simulink model "EV_0808_mohu"  (R2018a)
settings: Solver=VariableStepAuto  StartTime=0.0  StopTime=1370  RelTol=1e-3
undefined symbols (not defined in the file or in its folder): batt, cyc_spd, cyc_time, DiscIntNeverNeededParam, fr_effi, TIME_STEP, tm, UC, vcu, vehicle
libraries: simulink x9, fuzblock x1
(part 1 of 2)
settings Model: Creator=FlowerCater  LastModifiedBy=FlowerCater
settings SolverCC: ZeroCrossAlgorithm=Adaptive
settings DebuggingCC: MaxConsecutiveZCsMsg=none
settings CodeAppCC: StateflowObjectComments=on

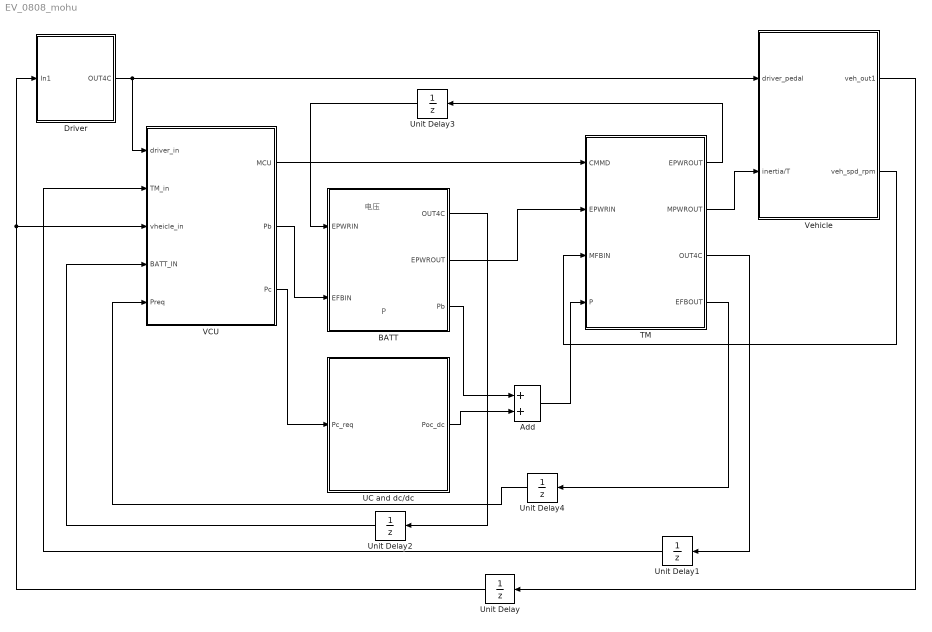
== system EV_0808_mohu ==
  note: 电压
  note: P
  Add : Sum
  BATT : Subsystem
  Driver : Subsystem
  TM : Subsystem
  UC and dc/dc : Subsystem
  Unit Delay : UnitDelay  SampleTime=-1
  Unit Delay1 : UnitDelay  SampleTime=-1
  Unit Delay2 : UnitDelay  SampleTime=-1
  Unit Delay3 : UnitDelay  InitialCondition=590  SampleTime=-1
  Unit Delay4 : UnitDelay  InitialCondition=590  SampleTime=-1
  VCU : Subsystem
  Vehicle : Subsystem
  wires:
  TM/4(EFBOUT) -> Unit Delay4/1
  Unit Delay1/1 -> VCU/2(TM_in)
  Unit Delay2/1 -> VCU/4(BATT_IN)
  TM/2(MPWROUT) -> Vehicle/2(inertia/T)
  TM/1(EPWROUT) -> Unit Delay3/1
  Driver/1(OUT4C) -> VCU/1(driver_in), Vehicle/1(driver_pedal)
  Unit Delay/1 -> Driver/1(In1), VCU/3(vheicle_in)
  Unit Delay3/1 -> BATT/1(EPWRIN)
  BATT/2(EPWROUT) -> TM/2(EPWRIN)
  BATT/1(OUT4C) -> Unit Delay2/1
  VCU/3(Pc) -> UC and dc/dc/1(Pc_req)
  Add/1 -> TM/4(P)
  UC and dc/dc/1(Poc_dc) -> Add/2
  Vehicle/2(veh_spd_rpm) -> TM/3(MFBIN)
  Unit Delay4/1 -> VCU/5(Preq)
  VCU/2(Pb) -> BATT/2(EFBIN)
  VCU/1(MCU) -> TM/1(CMMD)
  BATT/3(Pb) -> Add/1
  TM/3(OUT4C) -> Unit Delay1/1
  Vehicle/1(veh_out1) -> Unit Delay/1

== system EV_0808_mohu/BATT ==
  note: batt_loss_kw
  note: batt_soc
  EPWRIN : Inport
  EFBIN : Inport  Port=2
  Battery degradation : Subsystem
  Bus Creator : BusCreator  Inputs=2
  Bus Creator2 : BusCreator  Inputs=10
  Bus Selector : BusSelector  OutputSignals=V_Volt_v
  Constant2 : Constant  Value=25
  Derice SOC : Subsystem
  Divide1 : Product  Inputs=/*
  Internal Heating : Subsystem
  Product : Product
  Saturation : Saturate  UpperLimit=250  LowerLimit=-200
  batt_curr : Scope
  batt_curra : Scope
  batt_soc : Scope
  batt_v : Scope
  max power limitation : Subsystem
  output voltage : Subsystem
  resistance and voltage : Subsystem
  OUT4C : Outport  InitialOutput=0
  EPWROUT : Outport  Port=2  InitialOutput=0
  Pb : Outport  Port=3
  tag scope: Ub=global
  wires:
  output voltage/2(batt_volt_drop_v) -> Internal Heating/3(lost_volt_v)
  Derice SOC/2(ah_throughout_ahrs) -> resistance and voltage/3(ah_throughout_ahrs), Battery degradation/2(DR), Bus Creator2/9  "batt_throughout_ah"
  output voltage/1(batt_out_volt_v) -> batt_v/1, Bus Creator2/2, [Ub], Bus Creator/1  "V_Volt_v"
  Derice SOC/1(batt_soc) -> Bus Creator2/6, Bus Creator/2, max power limitation/3(batt_soc), Battery degradation/1(SOC), batt_soc/1, resistance and voltage/2(batt_soc)  "batt_soc"
  max power limitation/1(dischar_peak_pwr_kw) -> Bus Creator2/7  "dischar_peak_pwr_kw"
  Bus Creator/1 -> EPWROUT/1
  resistance and voltage/1(batt_oc_volt_v) -> max power limitation/1(batt_volt_oc_v), output voltage/1(battery_oc_volt_v)
  max power limitation/2(char_peak_pwr_kw) -> Bus Creator2/8  "char_peak_pwr_kw"
  Derice SOC/3(batt_curr_amp) -> resistance and voltage/4(current_amp), Bus Creator2/3, Product/2, Saturation/1, Internal Heating/2(Curr_amp), output voltage/2(batt_curr_amp)  "V_Curr_amp"
  Constant2/1 -> Internal Heating/1(amb_temp_degc)
  resistance and voltage/2(batt_res_ohm) -> max power limitation/2(batt_res_ohm), Bus Creator2/5, output voltage/3(battery_res_ohms)  "batt_res_ohm"
  Internal Heating/2(batt_temp_degc) -> resistance and voltage/1(temp_degc), max power limitation/4(batt_temp_degc), Bus Creator2/4  "batt_temp_degc"
  EPWRIN/1 -> Bus Selector/1
  Bus Selector/1 -> Derice SOC/1(EPWRIN), Divide1/1  "<V_Volt_v>"
  Bus Creator2/1 -> OUT4C/1
  Internal Heating/1(batt_pwr_lose_kw) -> Bus Creator2/10
  Saturation/1 -> Product/1, batt_curra/1
  Divide1/1 -> batt_curr/1, Derice SOC/2(EFBIN)
  Product/1 -> Pb/1
  EFBIN/1 -> Divide1/2
  Battery degradation/1(aging) -> Bus Creator2/1

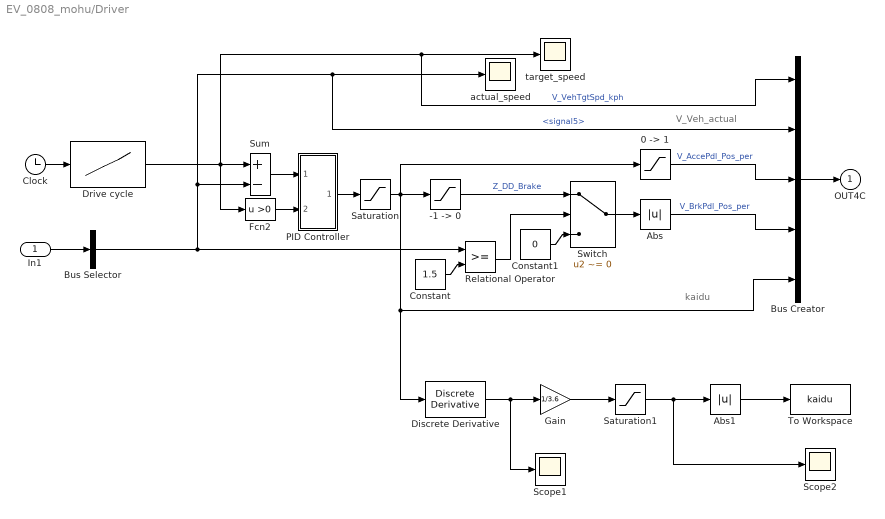
== system EV_0808_mohu/Driver ==
  note: V_Veh_actual
  note: kaidu
  In1 : Inport
  "-1 -> 0" : Saturate  UpperLimit=0  LowerLimit=-1
  "0 -> 1 " : Saturate  UpperLimit=1  LowerLimit=0
  Abs : Abs  SaturateOnIntegerOverflow=on
  Abs1 : Abs
  Bus Creator : BusCreator  Inputs=5
  Bus Selector : BusSelector  OutputSignals=signal5
  Clock : Clock
  Constant : Constant  Value=1.5
  Constant1 : Constant  Value=0
  Discrete Derivative : simulink/Discrete/Discrete Derivative  gainval=1.0  ICPrevScaledInput=0.0  OutMin=[]  OutMax=[]  OutDataType=fixdt(1, 16)  OutScaling=2^-10  DoSatur=off
  "Drive cycle " : Lookup  InputValues=cyc_time  Table=cyc_spd  SaturateOnIntegerOverflow=on
  Fcn2 : Fcn  Expr=u >0
  Gain : Gain  Gain=1/3.6
  PID Controller : Subsystem  mask(PID Controller){P=1, I=0.001, D=0, initial=0, max=1, min=-1}
      mask prompts: P "Proportional:"; I "Integral:"; D "Derivative:"; initial "Initial value"; max "Range max value"; min "Range min value"
      mask help:
      | Enter expressions for proportional, integral, and derivative terms.
      | P+I/s+Ds
      mask Help: This block implements a PID controller where parameters are entered for the Proportional, Integral and Derivative terms. Unmask this block to see how it works. The derivative term is implemented using a true derivative block.
      mask Display: disp('PID')
  Relational Operator : RelationalOperator  OutDataTypeStr=boolean  RndMeth=Nearest
  Saturation : Saturate  UpperLimit=1  LowerLimit=-1
  Saturation1 : Saturate  UpperLimit=1  LowerLimit=-1
  Scope1 : Scope
  Scope2 : Scope
  Sum : Sum  Inputs=+-  SaturateOnIntegerOverflow=on
  Switch : Switch  Criteria=u2 ~= 0
  To Workspace : ToWorkspace  VariableName=kaidu  SaveFormat=Timeseries  SampleTime=-1
  actual_speed : Scope
  target_speed : Scope
  OUT4C : Outport  InitialOutput=0
  wires:
  Bus Creator/1 -> OUT4C/1
  Fcn2/1 -> PID Controller/2(reset)
  Bus Selector/1 -> Bus Creator/2, actual_speed/1, Sum/2, Relational Operator/1  "<signal5>"
  Sum/1 -> PID Controller/1(In_1)
  Constant/1 -> Relational Operator/2
  Relational Operator/1 -> Switch/2
  Constant1/1 -> Switch/3
  PID Controller/1(Out_1) -> Saturation/1
  Switch/1 -> Abs/1
  "-1 -> 0"/1 -> Switch/1  "Z_DD_Brake"
  Clock/1 -> "Drive cycle "/1
  "Drive cycle "/1 -> Fcn2/1, Bus Creator/1, target_speed/1, Sum/1  "V_VehTgtSpd_kph"
  Saturation/1 -> "-1 -> 0"/1, "0 -> 1 "/1, Bus Creator/5, Discrete Derivative/1
  Abs/1 -> Bus Creator/4  "V_BrkPdl_Pos_per"
  "0 -> 1 "/1 -> Bus Creator/3  "V_AccePdl_Pos_per"
  In1/1 -> Bus Selector/1
  Discrete Derivative/1 -> Scope1/1, Gain/1
  Abs1/1 -> To Workspace/1
  Saturation1/1 -> Scope2/1, Abs1/1
  Gain/1 -> Saturation1/1

== system EV_0808_mohu/TM ==
  note: 电池动力输入
  note: 电机转动惯量
  CMMD : Inport
  EPWRIN : Inport  Port=2
  MFBIN : Inport  Port=3
  P : Inport  Port=4
  Bus Creator : BusCreator  Inputs=5
  Bus Creator1 : BusCreator  Inputs=1
  Bus Creator2 : BusCreator  Inputs=2
  Bus Selector : BusSelector  OutputSignals=V_BrkTq_Req_nm
  Bus Selector1 : BusSelector  OutputSignals=signal1
  Bus Selector2 : BusSelector  OutputSignals=V_Volt_v,batt_soc
  Constant : Constant  Value=tm.inertia
  Current Generation : Subsystem
  Intenal Heating : Subsystem
  Terminator : Terminator
  Terminator1 : Terminator
  Torque management : Subsystem
  Unit Delay1 : UnitDelay  SampleTime=-1
  EPWROUT : Outport
  MPWROUT : Outport  Port=2
  OUT4C : Outport  Port=3
  EFBOUT : Outport  Port=4
  wires:
  Constant/1 -> Bus Creator2/2  "tm.inertia"
  Current Generation/2(motor_eff_per) -> Terminator/1
  Torque management/1(" torque_req_nm") -> Bus Creator/4, Bus Creator2/1, Current Generation/1(torque_req_nm)  "V_Actual_BrkTq_nm"
  Current Generation/3(pwr_loss_w) -> Bus Creator/5, Intenal Heating/1(pwr_loss_w)  "TM_loss_W"
  EPWRIN/1 -> Bus Selector2/1
  CMMD/1 -> Bus Selector/1
  Bus Selector/1 -> Torque management/1(tq_req_nm)  "<V_BrkTq_Req_nm>"
  Bus Creator2/1 -> MPWROUT/1
  MFBIN/1 -> Unit Delay1/1
  Current Generation/1(motor_curr_amp) -> Bus Creator/3  "V_CurrDCamp"
  Intenal Heating/1(cool_temp_degc) -> Bus Creator/1, Torque management/3(cool_temp_degc)  "V_Cool_Temp_degc"
  Bus Creator/1 -> OUT4C/1
  Unit Delay1/1 -> Bus Selector1/1
  Bus Selector1/1 -> Current Generation/2(motor_spd_rpm), Torque management/4(motor_spd_rpm), Bus Creator/2  "<signal1>"
  Bus Selector2/1 -> Current Generation/3(volt_v), Bus Creator1/1  "<V_Volt_v>"
  Bus Creator1/1 -> EPWROUT/1
  Bus Selector2/2 -> Torque management/2(soc)  "<batt_soc>"
  Current Generation/4(P) -> EFBOUT/1  "p"
  P/1 -> Terminator1/1

== system EV_0808_mohu/UC and dc//dc ==
  Pc_req : Inport
  Gain : Gain  Gain=-1
  Memory : Memory
  Pcdc : Scope
  Product1 : Product
  Switch : Switch  Criteria=u2 > Threshold
  UC : Subsystem
  charge : Lookup_n-D  BreakpointsForDimension1=[0:2000:8000]  BreakpointsForDimension2=[0.2:0.2:1]  Table=[0.8 0.8 0.8 0.8 0.8;0.945 0.952 0.965 0.972 0.977;0.94 0.95 0.957 0.965 0.97;0.938 0.946 0.952 0.962 0.964;0.934 0.944 0.95 0.96 0.962]  InternalRulePriority=Speed  RndMeth=Simplest  InputSameDT=on
  discharge : Lookup_n-D  BreakpointsForDimension1=[0:2000:8000]  BreakpointsForDimension2=[0.2:0.2:1]  Table=[0.8 0.8 0.8 0.8 0.8;0.945 0.952 0.965 0.972 0.977;0.94 0.95 0.957 0.965 0.97;0.938 0.946 0.952 0.962 0.964;0.934 0.944 0.95 0.96 0.962]  InternalRulePriority=Speed  RndMeth=Simplest  InputSameDT=on
  电压比 : Product  Inputs=/*
  电压比1 : Product  Inputs=*/
  Poc_dc : Outport
  wires:
  电压比1/1 -> Switch/1
  电压比/1 -> Memory/1
  UC/1(Pc) -> 电压比1/1, Product1/1, Switch/2, discharge/1, Gain/1
  charge/1 -> Product1/2
  discharge/1 -> 电压比1/2
  Gain/1 -> charge/1
  [Uc] -> 电压比/1
  Product1/1 -> Switch/3
  Memory/1 -> discharge/2, charge/2
  [Ub] -> 电压比/2
  Switch/1 -> Pcdc/1, Poc_dc/1
  Pc_req/1 -> UC/1(Pc-req (W))

== system EV_0808_mohu/VCU ==
  driver_in : Inport
  TM_in : Inport  Port=2
  vheicle_in : Inport  Port=3
  BATT_IN : Inport  Port=4
  Preq : Inport  Port=5
  Bus Creator2 : BusCreator  Inputs=5
  Display : Display
  Gain : Gain
  Gain1 : Gain
  Gain2 : Gain
  Subsystem1 : Subsystem
  Subsystem3 : Subsystem
  To Workspace : ToWorkspace  VariableName=tm_act_tq11  SampleTime=-1
      settings: MaxDataPoints=Inf
  To Workspace1 : ToWorkspace  VariableName=tm_act_spd  SampleTime=-1
      settings: MaxDataPoints=Inf
  controller : Subsystem
  max generation  torque : Lookup  InputValues=tm.max_gen_tq_x_rpm  Table=tm.max_gen_tq_y_nm  LookUpMeth=Interpolation-Use End Values
  max motoring torque : Lookup  InputValues=tm.max_mot_tq_x_rpm  Table=tm.max_mot_tq_y_nm  LookUpMeth=Interpolation-Use End Values
  续驶里程估计 : Subsystem
  能耗计算 : Subsystem
  MCU : Outport
  Pb : Outport  Port=2
  Pc : Outport  Port=3
  wires:
  Gain/1 -> Bus Creator2/1  "V_BrkTq_Req_nm"
  max motoring torque/1 -> Bus Creator2/2  "V_MaxMotTq_nm"
  max generation  torque/1 -> Bus Creator2/3  "V_MaxGenTq_nm"
  Gain1/1 -> Bus Creator2/4, To Workspace1/1  "V_Spd_rpm"
  Gain2/1 -> Bus Creator2/5, To Workspace/1  "V_ActBrkTq_nm"
  Bus Creator2/1 -> MCU/1
  Subsystem1/1(V_Spd_rmp) -> Subsystem3/1(V_Spd_rpm), max motoring torque/1, Gain1/1, max generation  torque/1
  TM_in/1 -> 能耗计算/2(In3), Subsystem1/1(TM_in)
  driver_in/1 -> 能耗计算/1(In1), Subsystem1/2(Dri_in)
  vheicle_in/1 -> 续驶里程估计/2(veh_in), Subsystem1/3(vheicle_in), 能耗计算/3(In2)
  BATT_IN/1 -> 续驶里程估计/1(batt_in), 能耗计算/4(In4)
  Subsystem1/2(rotor drive torque available nm) -> Gain2/1
  Subsystem3/1(TM_TqReq_nm) -> Gain/1
  Subsystem1/3(Tq_Req_nm) -> Subsystem3/2(dri_TqReq_nm)
  能耗计算/1(E_FS) -> Display/1
  Preq/1 -> controller/1(Preq (W))
  controller/1(Pb (W)) -> Pb/1
  controller/2(Pc (W)) -> Pc/1

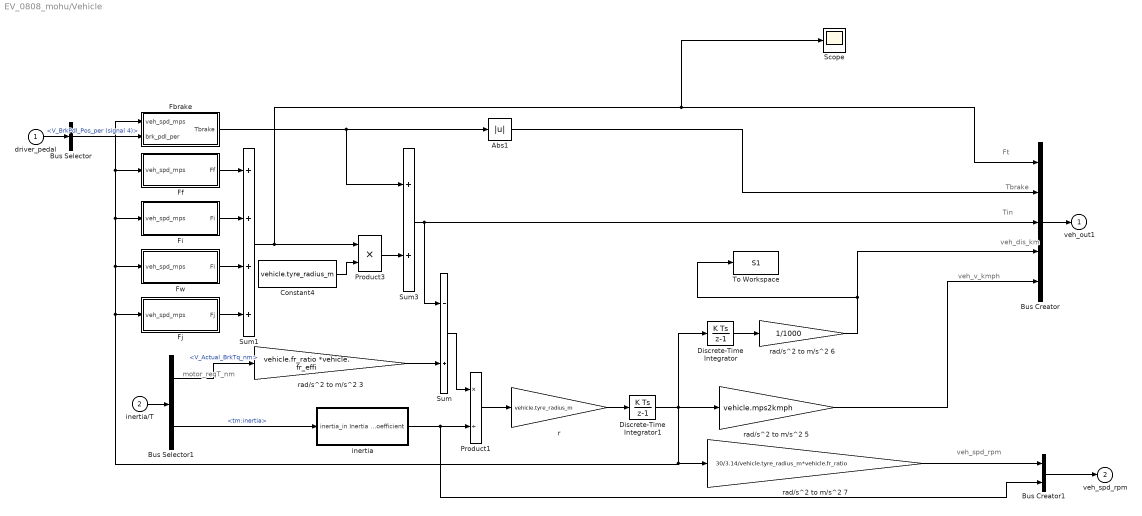
== system EV_0808_mohu/Vehicle ==
  note: veh_spd_rpm
  note: veh_v_kmph
  note: veh_dis_km
  note: Tin
  note: Tbrake
  note: Ft
  note: motor_reqT_nm
  driver_pedal : Inport
  inertia/T : Inport  Port=2
  Abs1 : Abs
  Bus Creator : BusCreator  Inputs=5
  Bus Creator1 : BusCreator  Inputs=2
  Bus Selector : BusSelector  OutputSignals=V_BrkPdl_Pos_per (signal 4)
  Bus Selector1 : BusSelector  OutputSignals=V_Actual_BrkTq_nm,tm:inertia
  Constant4 : Constant  Value=vehicle.tyre_radius_m
  Discrete-Time Integrator : DiscreteIntegrator  SampleTime=0.01  ICPrevOutput=DiscIntNeverNeededParam  ICPrevScaledInput=DiscIntNeverNeededParam
  Discrete-Time Integrator1 : DiscreteIntegrator  SampleTime=0.01  LimitOutput=on  LowerSaturationLimit=0  ICPrevOutput=DiscIntNeverNeededParam  ICPrevScaledInput=DiscIntNeverNeededParam
  Fbrake : Subsystem
  Ff : Subsystem
  Fi : Subsystem
  Fj : Subsystem
  Fw : Subsystem
  Product1 : Product  Inputs=*/  SaturateOnIntegerOverflow=on  OutDataTypeStr=Inherit: Same as first input
  Product3 : Product  SaturateOnIntegerOverflow=on  InputSameDT=on  OutDataTypeStr=Inherit: Same as first input
  Scope : Scope
  Sum : Sum  Inputs=-+  SaturateOnIntegerOverflow=on
  Sum1 : Sum  Inputs=++++  SaturateOnIntegerOverflow=on  InputSameDT=on  OutDataTypeStr=Inherit: Same as first input
  Sum3 : Sum  SaturateOnIntegerOverflow=on  InputSameDT=on  OutDataTypeStr=Inherit: Same as first input
  To Workspace : ToWorkspace  VariableName=S1  SampleTime=-1
  inertia : Subsystem
  r : Gain  Gain=vehicle.tyre_radius_m  SaturateOnIntegerOverflow=on  OutDataTypeStr=Inherit: Same as input  ParamDataTypeStr=Inherit: Same as input
  rad/s^2 to m/s^2 3 : Gain  Gain=vehicle.fr_ratio *vehicle. fr_effi  SaturateOnIntegerOverflow=on  OutDataTypeStr=Inherit: Same as input  ParamDataTypeStr=Inherit: Same as input
  rad/s^2 to m/s^2 5 : Gain  Gain=vehicle.mps2kmph  SaturateOnIntegerOverflow=on  OutDataTypeStr=Inherit: Same as input  ParamDataTypeStr=Inherit: Same as input
  rad/s^2 to m/s^2 6 : Gain  Gain=1/1000  SaturateOnIntegerOverflow=on  OutDataTypeStr=Inherit: Same as input  ParamDataTypeStr=Inherit: Same as input
  rad/s^2 to m/s^2 7 : Gain  Gain=30/3.14/vehicle.tyre_radius_m*vehicle.fr_ratio  SaturateOnIntegerOverflow=on  OutDataTypeStr=Inherit: Same as input  ParamDataTypeStr=Inherit: Same as input
  veh_out1 : Outport  InitialOutput=0
  veh_spd_rpm : Outport  Port=2  InitialOutput=0
  wires:
  driver_pedal/1 -> Bus Selector/1
  Ff/1(Ff) -> Sum1/1
  Fi/1(Fi) -> Sum1/2
  Fw/1(Fi) -> Sum1/3
  Fj/1(Fj) -> Sum1/4
  Sum1/1 -> Scope/1, Bus Creator/1, Product3/1
  Constant4/1 -> Product3/2
  Product3/1 -> Sum3/2
  Fbrake/1(Tbrake) -> Abs1/1, Sum3/1
  Abs1/1 -> Bus Creator/2
  rad/s^2 to m/s^2 3/1 -> Sum/2
  Sum3/1 -> Bus Creator/3, Sum/1
  Bus Selector/1 -> Fbrake/2(brk_pdl_per)  "<V_BrkPdl_Pos_per (signal 4)>"
  inertia/1(Inertia coefficient) -> Bus Creator1/2, Product1/2
  Sum/1 -> Product1/1
  Product1/1 -> r/1
  r/1 -> Discrete-Time Integrator1/1
  Bus Selector1/2 -> inertia/1(inertia_in)  "<tm:inertia>"
  Discrete-Time Integrator1/1 -> Fbrake/1(veh_spd_mps), Ff/1(veh_spd_mps), Fi/1(veh_spd_mps), Fw/1(veh_spd_mps), Fj/1(veh_spd_mps), rad/s^2 to m/s^2 7/1, Discrete-Time Integrator/1, rad/s^2 to m/s^2 5/1
  rad/s^2 to m/s^2 5/1 -> Bus Creator/5
  rad/s^2 to m/s^2 7/1 -> Bus Creator1/1
  rad/s^2 to m/s^2 6/1 -> Bus Creator/4, To Workspace/1
  Discrete-Time Integrator/1 -> rad/s^2 to m/s^2 6/1
  inertia/T/1 -> Bus Selector1/1
  Bus Creator/1 -> veh_out1/1
  Bus Creator1/1 -> veh_spd_rpm/1
  Bus Selector1/1 -> rad/s^2 to m/s^2 3/1  "<V_Actual_BrkTq_nm>"

== system EV_0808_mohu/BATT/Battery degradation ==
  note: 额定容量
  SOC : Inport
  DR : Inport  Port=2
  Add3 : Sum  Inputs=++++
  Constant1 : Constant  Value=120
  Constant3 : Constant  Value=0.069
  Constant4 : Constant  Value=21.714
  Divide : Product  Inputs=*/
  Fcn : Fcn  Expr=-0.573*u+0.004*(u^2)
  Fcn1 : Fcn  Expr=3.13*u-2.34*(u^2)
  Product1 : Product  Inputs=3
  aging : Outport
  wires:
  SOC/1 -> Product1/1, Fcn/1
  Divide/1 -> Product1/3, Fcn1/1
  Constant4/1 -> Add3/4
  Fcn1/1 -> Add3/3
  Fcn/1 -> Add3/1
  Product1/1 -> Add3/2
  Constant3/1 -> Product1/2
  Add3/1 -> aging/1
  Constant1/1 -> Divide/2
  DR/1 -> Divide/1

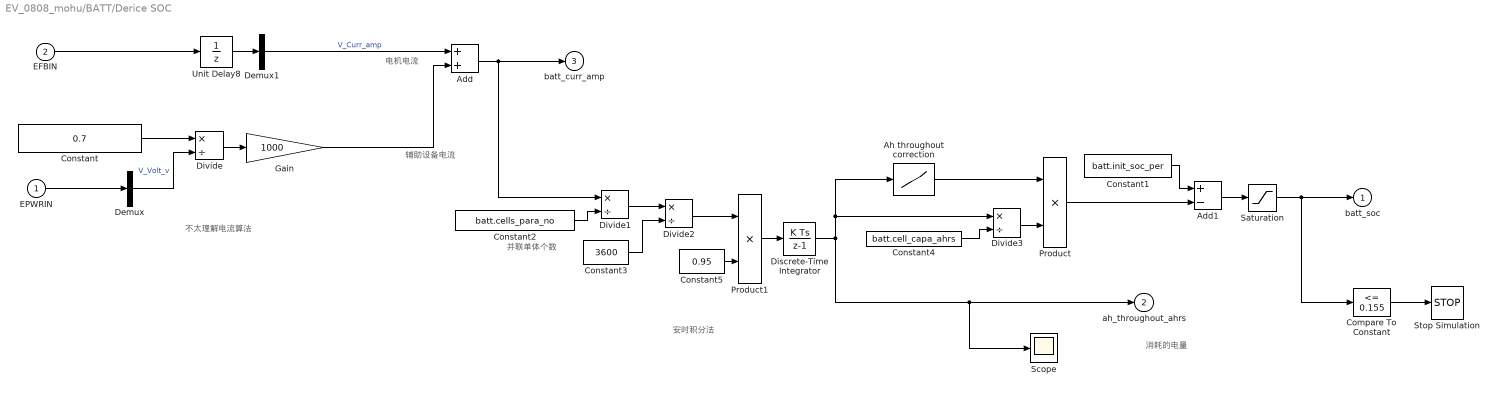
== system EV_0808_mohu/BATT/Derice SOC ==
  note: 安时积分法
  note: 消耗的电量
  note: 并联单体个数
  note: 不太理解电流算法
  note: 辅助设备电流
  note: 电机电流
  EPWRIN : Inport
  EFBIN : Inport  Port=2
  Add : Sum
  Add1 : Sum  Inputs=+-
  Ah throughout correction : Lookup  InputValues=batt.energy_deter_x_brkthrough_ahrs  Table=batt.energy_deter_y  LookUpMeth=Interpolation-Use End Values
  Compare To Constant : simulink/Logic and Bit Operations/Compare To Constant  relop=<=  const=0.155  OutDataTypeStr=boolean
  Constant : Constant  Value=0.7
  Constant1 : Constant  Value=batt.init_soc_per
  Constant2 : Constant  Value=batt.cells_para_no
  Constant3 : Constant  Value=3600
  Constant4 : Constant  Value=batt.cell_capa_ahrs
  Constant5 : Constant  Value=0.95
  Demux : Demux  Outputs=1
  Demux1 : Demux  Outputs=1
  Discrete-Time Integrator : DiscreteIntegrator  SampleTime=0.01  ICPrevOutput=DiscIntNeverNeededParam  ICPrevScaledInput=DiscIntNeverNeededParam
  Divide{,1..3} (4 alike) : Product  Inputs=*/
  Gain : Gain  Gain=1000
  Product : Product
  Product1 : Product
  Saturation : Saturate  UpperLimit=1  LowerLimit=0
  Scope : Scope
  Stop Simulation : Stop
  Unit Delay8 : UnitDelay  SampleTime=-1
  batt_soc : Outport  InitialOutput=0
  ah_throughout_ahrs : Outport  Port=2  InitialOutput=0
  batt_curr_amp : Outport  Port=3  InitialOutput=0
  wires:
  Product/1 -> Add1/2
  Constant1/1 -> Add1/1
  Divide3/1 -> Product/2
  Ah throughout correction/1 -> Product/1
  Add1/1 -> Saturation/1
  EFBIN/1 -> Unit Delay8/1
  Unit Delay8/1 -> Demux1/1
  Constant/1 -> Divide/1
  Demux/1 -> Divide/2  "V_Volt_v"
  EPWRIN/1 -> Demux/1
  Demux1/1 -> Add/1  "V_Curr_amp"
  Gain/1 -> Add/2
  Divide/1 -> Gain/1
  Constant2/1 -> Divide1/2
  Constant3/1 -> Divide2/2
  Constant4/1 -> Divide3/2
  Divide1/1 -> Divide2/1
  Discrete-Time Integrator/1 -> Ah throughout correction/1, Divide3/1, Scope/1, ah_throughout_ahrs/1
  Divide2/1 -> Product1/1
  Constant5/1 -> Product1/2
  Add/1 -> Divide1/1, batt_curr_amp/1
  Product1/1 -> Discrete-Time Integrator/1
  Saturation/1 -> Compare To Constant/1, batt_soc/1
  Compare To Constant/1 -> Stop Simulation/1

== system EV_0808_mohu/BATT/Internal Heating ==
  note: 电池损失功率
  amb_temp_degc : Inport
  Curr_amp : Inport  Port=2
  lost_volt_v : Inport  Port=3
  1/thermal capacity : Gain  Gain=1/(batt.thermal_capa_jpk*batt.cells_para_no*batt.cells_series_no)  SaturateOnIntegerOverflow=on  OutDataTypeStr=Inherit: Same as input  ParamDataTypeStr=Inherit: Same as input
  1/thermal resistance : Gain  Gain=batt.thermal_disp_wpk  SaturateOnIntegerOverflow=on  OutDataTypeStr=Inherit: Same as input  ParamDataTypeStr=Inherit: Same as input
  Abs : Abs  SaturateOnIntegerOverflow=on
  Discrete-Time Integrator1 : DiscreteIntegrator  SampleTime=0.01  LimitOutput=on  LowerSaturationLimit=0  ICPrevOutput=DiscIntNeverNeededParam  ICPrevScaledInput=DiscIntNeverNeededParam
  Gain1 : Gain  Gain=1/1000
  Product1 : Product  SaturateOnIntegerOverflow=on  InputSameDT=on  OutDataTypeStr=Inherit: Same as first input
  Sum1 : Sum  Inputs=+-  SaturateOnIntegerOverflow=on  InputSameDT=on  OutDataTypeStr=Inherit: Same as first input
  Sum2 : Sum  Inputs=+-  SaturateOnIntegerOverflow=on  InputSameDT=on  OutDataTypeStr=Inherit: Same as first input
  To Workspace : ToWorkspace  VariableName=batt_temp_degc  SaveFormat=Timeseries  SampleTime=-1
  batt_pwr_lose_kw : Outport  InitialOutput=0
  batt_temp_degc : Outport  Port=2  InitialOutput=0
  wires:
  Gain1/1 -> batt_pwr_lose_kw/1
  Sum2/1 -> 1/thermal resistance/1
  amb_temp_degc/1 -> Sum2/2
  Product1/1 -> Abs/1
  Abs/1 -> Gain1/1, Sum1/1
  Sum1/1 -> 1/thermal capacity/1
  1/thermal resistance/1 -> Sum1/2
  Curr_amp/1 -> Product1/1
  lost_volt_v/1 -> Product1/2
  1/thermal capacity/1 -> Discrete-Time Integrator1/1
  Discrete-Time Integrator1/1 -> To Workspace/1, batt_temp_degc/1, Sum2/1

== system EV_0808_mohu/BATT/max power limitation ==
  note: 负值取小
  note: 正值取大
  note: 实际充电峰值功率
  note: 实际放电峰值功率
  note: 充电峰值功率
  note: 放电峰值功率
  batt_volt_oc_v : Inport
  batt_res_ohm : Inport  Port=2
  batt_soc : Inport  Port=3
  batt_temp_degc : Inport  Port=4
  MinMax1 : MinMax  Inputs=2  SaturateOnIntegerOverflow=on  InputSameDT=on
  MinMax2 : MinMax  Function=max  Inputs=2  SaturateOnIntegerOverflow=on  InputSameDT=on
  Pack Peak Discharging Power : Lookup2D  RowIndex=batt.max_discharge_pwr_x_soc_per  ColumnIndex=batt.max_discharge_pwr_y_temp_degc  Table=batt.max_discharge_pwr_z_kw  LookUpMeth=Interpolation-Use End Values  SaturateOnIntegerOverflow=on  InputSameDT=on
  Pack peak charging power : Lookup2D  RowIndex=batt.max_charge_pwr_x_soc_per  ColumnIndex=batt.max_charge_pwr_y_temp_degc  Table=batt.max_charge_pwr_z_kw  LookUpMeth=Interpolation-Use End Values  SaturateOnIntegerOverflow=on  InputSameDT=on
  peak chrg power : Subsystem
  peak dischrg power : Subsystem
  dischar_peak_pwr_kw : Outport
  char_peak_pwr_kw : Outport  Port=2
  wires:
  peak chrg power/1(chrg_peak_pwr_kw) -> MinMax2/2
  batt_res_ohm/1 -> peak chrg power/1(batt_res_ohms), peak dischrg power/1(batt_res_ohms)
  MinMax2/1 -> char_peak_pwr_kw/1
  MinMax1/1 -> dischar_peak_pwr_kw/1
  Pack Peak Discharging Power/1 -> MinMax1/1
  Pack peak charging power/1 -> MinMax2/1  "Charge acceptance (<0)"
  peak dischrg power/1(dischrg_peak_pwr_kw) -> MinMax1/2
  batt_volt_oc_v/1 -> peak chrg power/2(batt_oc_volt_v), peak dischrg power/2(batt_oc_volt_v)
  batt_soc/1 -> Pack Peak Discharging Power/1, Pack peak charging power/1
  batt_temp_degc/1 -> Pack Peak Discharging Power/2, Pack peak charging power/2

== system EV_0808_mohu/BATT/output voltage ==
  note: 损失电压
  note: 输出端电压
  battery_oc_volt_v : Inport
  batt_curr_amp : Inport  Port=2
  battery_res_ohms : Inport  Port=3
  Add : Sum  Inputs=+-
  Product : Product
  batt_out_volt_v : Outport  InitialOutput=0
  batt_volt_drop_v : Outport  Port=2  InitialOutput=0
  wires:
  batt_curr_amp/1 -> Product/2
  Product/1 -> batt_volt_drop_v/1, Add/2
  battery_oc_volt_v/1 -> Add/1
  battery_res_ohms/1 -> Product/1
  Add/1 -> batt_out_volt_v/1

== system EV_0808_mohu/BATT/resistance and voltage ==
  note: 根据电量消耗对内阻的修正
  note: 欧姆内阻
  note: 放电电流为正
  note: 电池开路电压
  temp_degc : Inport
  batt_soc : Inport  Port=2
  ah_throughout_ahrs : Inport  Port=3
  current_amp : Inport  Port=4
  Add : Sum
  Constant : Constant  Value=1.0
  Constant1 : Constant  Value=0
  N_series : Gain  Gain=batt.cells_series_no  SaturateOnIntegerOverflow=on  OutDataTypeStr=Inherit: Same as input  ParamDataTypeStr=Inherit: Same as input
  N_series/ N_parallel : Gain  Gain=batt.cells_series_no/batt.cells_para_no  SaturateOnIntegerOverflow=on  OutDataTypeStr=Inherit: Same as input  ParamDataTypeStr=Inherit: Same as input
  Open Circuit Voltage : Lookup2D  RowIndex=batt.cell_open_volt_x_soc_per  ColumnIndex=batt.cell_open_volt_y_degc  Table=batt.cell_open_volt_z_v  LookUpMeth=Interpolation-Use End Values  SaturateOnIntegerOverflow=on  InputSameDT=on
  Product : Product  SaturateOnIntegerOverflow=on  InputSameDT=on  OutDataTypeStr=Inherit: Same as first input
  Product1 : Product
  Relational Operator : RelationalOperator  OutDataTypeStr=boolean  RndMeth=Nearest
  Switch : Switch  Criteria=u2 ~= 0
  To Workspace : ToWorkspace  VariableName=Pd1  SampleTime=-1
  ah throughout correction : Lookup  InputValues=batt.resis_deter_x_brkthrough_ahrs  Table=batt.resis_deter_y  LookUpMeth=Interpolation-Use End Values
  charge resistance table : Lookup2D  RowIndex=batt.resis_chrg_x_soc_per  ColumnIndex=batt.resis_chrg_y_temp_degc  Table=batt.resis_chrg_z_ohm  LookUpMeth=Interpolation-Use End Values  SaturateOnIntegerOverflow=on  InputSameDT=on
  discharge resistance table : Lookup2D  RowIndex=batt.resis_dischrg_x_soc_per  ColumnIndex=batt.resis_dischrg_y_temp_degc  Table=batt.resis_dischrg_z_ohm  LookUpMeth=Interpolation-Use End Values  SaturateOnIntegerOverflow=on  InputSameDT=on
  batt_oc_volt_v : Outport  InitialOutput=0
  batt_res_ohm : Outport  Port=2  InitialOutput=0
  wires:
  Add/1 -> Product/2
  Constant/1 -> Add/2
  ah throughout correction/1 -> Add/1
  ah_throughout_ahrs/1 -> ah throughout correction/1
  Product/1 -> batt_res_ohm/1
  N_series/ N_parallel/1 -> Product/1
  discharge resistance table/1 -> Switch/1
  N_series/1 -> Product1/1, batt_oc_volt_v/1
  Open Circuit Voltage/1 -> N_series/1
  batt_soc/1 -> Open Circuit Voltage/1, discharge resistance table/1, charge resistance table/1
  temp_degc/1 -> Open Circuit Voltage/2, discharge resistance table/2, charge resistance table/2
  current_amp/1 -> Product1/2, Relational Operator/1
  Constant1/1 -> Relational Operator/2
  Relational Operator/1 -> Switch/2
  charge resistance table/1 -> Switch/3
  Switch/1 -> N_series/ N_parallel/1
  Product1/1 -> To Workspace/1

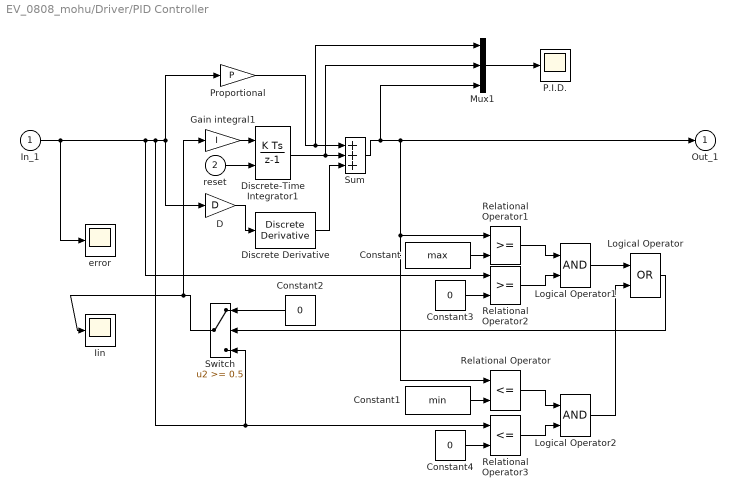
== system EV_0808_mohu/Driver/PID Controller ==
  In_1 : Inport
  reset : Inport  Port=2
  Constant : Constant  Value=max
  Constant1 : Constant  Value=min
  Constant2 : Constant  Value=0
  Constant3 : Constant  Value=0
  Constant4 : Constant  Value=0
  D : Gain  Gain=D  SaturateOnIntegerOverflow=on  OutDataTypeStr=Inherit: Same as input  ParamDataTypeStr=Inherit: Same as input
  Discrete Derivative : simulink/Discrete/Discrete Derivative  gainval=1.0  ICPrevScaledInput=0.0  InputProcessing=Inherited  OutMin=[]  OutMax=[]  OutDataType=fixdt(1, 16)  OutScaling=2^-10  DoSatur=off
  Discrete-Time Integrator1 : DiscreteIntegrator  InitialConditionSource=external  SampleTime=0.01  LimitOutput=on  LowerSaturationLimit=0  ICPrevOutput=DiscIntNeverNeededParam  ICPrevScaledInput=DiscIntNeverNeededParam
  Gain integral1 : Gain  Gain=I  SaturateOnIntegerOverflow=on  OutDataTypeStr=Inherit: Same as input  ParamDataTypeStr=Inherit: Same as input
  Iin : Scope
  Logical Operator : Logic  Operator=OR
  Logical Operator1 : Logic
  Logical Operator2 : Logic
  Mux1 : Mux  Inputs=3
  P.I.D. : Scope
  Proportional : Gain  Gain=P  SaturateOnIntegerOverflow=on  OutDataTypeStr=Inherit: Same as input  ParamDataTypeStr=Inherit: Same as input
  Relational Operator : RelationalOperator  Operator=<=  RndMeth=Nearest  InputSameDT=on
  Relational Operator1 : RelationalOperator  RndMeth=Nearest  InputSameDT=on
  Relational Operator2 : RelationalOperator  RndMeth=Nearest  InputSameDT=on
  Relational Operator3 : RelationalOperator  Operator=<=  RndMeth=Nearest  InputSameDT=on
  Sum : Sum  Inputs=+++  SaturateOnIntegerOverflow=on  InputSameDT=on  OutDataTypeStr=Inherit: Same as first input
  Switch : Switch  Threshold=0.5  SaturateOnIntegerOverflow=on  InputSameDT=on
  error : Scope
  Out_1 : Outport  InitialOutput=0
  wires:
  Logical Operator1/1 -> Logical Operator/1
  Logical Operator2/1 -> Logical Operator/2
  Relational Operator3/1 -> Logical Operator2/2
  Constant4/1 -> Relational Operator3/2
  Relational Operator/1 -> Logical Operator2/1
  Relational Operator2/1 -> Logical Operator1/2
  Constant3/1 -> Relational Operator2/2
  Constant1/1 -> Relational Operator/2
  Relational Operator1/1 -> Logical Operator1/1
  Constant/1 -> Relational Operator1/2
  Logical Operator/1 -> Switch/2
  Sum/1 -> Mux1/3, Relational Operator1/1, Relational Operator/1, Out_1/1
  In_1/1 -> Proportional/1, D/1, Relational Operator3/1, Switch/3, Relational Operator2/1, error/1
  Proportional/1 -> Mux1/1, Sum/1
  Constant2/1 -> Switch/1
  Switch/1 -> Gain integral1/1, Iin/1
  Discrete-Time Integrator1/1 -> Mux1/2, Sum/2
  D/1 -> Discrete Derivative/1
  Discrete Derivative/1 -> Sum/3
  reset/1 -> Discrete-Time Integrator1/2
  Gain integral1/1 -> Discrete-Time Integrator1/1
  Mux1/1 -> P.I.D./1

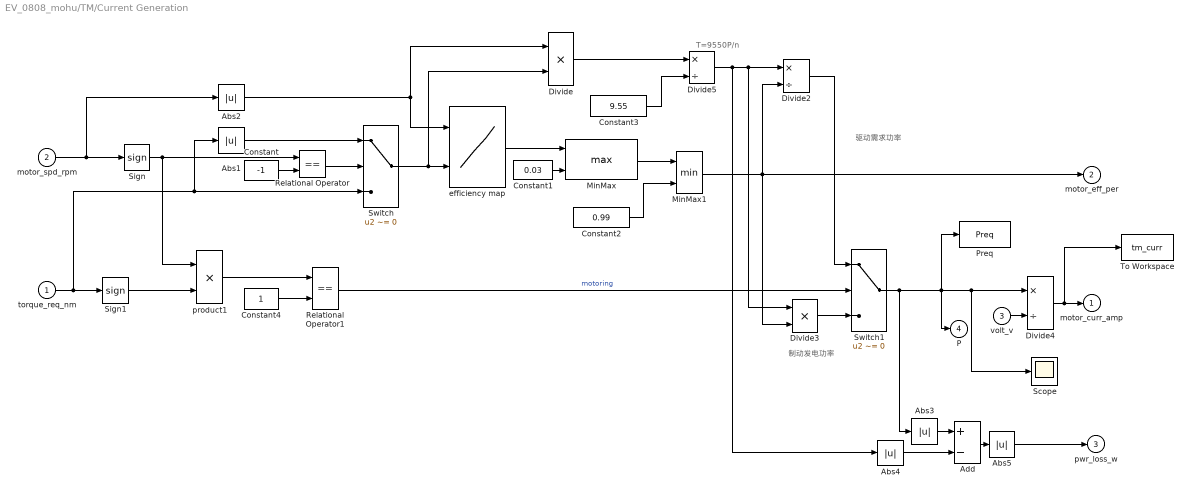
== system EV_0808_mohu/TM/Current Generation ==
  note: T=9550P/n
  note: 制动发电功率
  note: 驱动需求功率
  torque_req_nm : Inport
  motor_spd_rpm : Inport  Port=2
  volt_v : Inport  Port=3
  Abs{1..5} (5 alike) : Abs
  Add : Sum  Inputs=+-
  Constant : Constant  Value=-1  OutDataTypeStr=int8
  Constant1 : Constant  Value=0.03
  Constant2 : Constant  Value=0.99
  Constant3 : Constant  Value=9.55
  Constant4 : Constant  OutDataTypeStr=int8
  Divide : Product  Inputs=**
  Divide2 : Product  Inputs=*/
  Divide3 : Product  Inputs=**
  Divide4 : Product  Inputs=*/
  Divide5 : Product  Inputs=*/
  MinMax : MinMax  Function=max  Inputs=2
  MinMax1 : MinMax  Inputs=2
  Preq : ToWorkspace  VariableName=Preq  SampleTime=-1
      settings: Save2DSignal=2-D array (concatenate along first dimension)
  Relational Operator : RelationalOperator  Operator===  OutDataTypeStr=boolean  RndMeth=Nearest
  Relational Operator1 : RelationalOperator  Operator===  OutDataTypeStr=boolean  RndMeth=Nearest
  Scope : Scope
  Sign : Signum
  Sign1 : Signum
  Switch : Switch  Criteria=u2 ~= 0
  Switch1 : Switch  Criteria=u2 ~= 0
  To Workspace : ToWorkspace  VariableName=tm_curr  SampleTime=-1
      settings: Save2DSignal=2-D array (concatenate along first dimension)
  efficiency map : Lookup2D  RowIndex=tm.eff_x_rpm  ColumnIndex=tm.eff_y_nm  Table=tm.eff_z  LookUpMeth=Interpolation-Use End Values
  product1 : Product  Inputs=**
  motor_curr_amp : Outport  InitialOutput=0
  motor_eff_per : Outport  Port=2  InitialOutput=0
  pwr_loss_w : Outport  Port=3  InitialOutput=0
  P : Outport  Port=4  InitialOutput=0
  wires:
  Divide5/1 -> Divide2/1, Divide3/1, Abs4/1
  Constant3/1 -> Divide5/2
  Abs5/1 -> pwr_loss_w/1
  Add/1 -> Abs5/1
  Abs4/1 -> Add/2
  Abs3/1 -> Add/1
  Divide4/1 -> To Workspace/1, motor_curr_amp/1
  volt_v/1 -> Divide4/2
  Divide3/1 -> Switch1/3
  Divide2/1 -> Switch1/1
  MinMax1/1 -> Divide3/2, motor_eff_per/1, Divide2/2
  Divide/1 -> Divide5/1
  Abs2/1 -> efficiency map/1, Divide/1
  Switch/1 -> efficiency map/2, Divide/2
  Constant2/1 -> MinMax1/2
  MinMax/1 -> MinMax1/1
  Constant1/1 -> MinMax/2
  efficiency map/1 -> MinMax/1
  Abs1/1 -> Switch/1
  Relational Operator/1 -> Switch/2
  Constant/1 -> Relational Operator/2
  Relational Operator1/1 -> Switch1/2  "motoring"
  Sign1/1 -> product1/2
  Sign/1 -> product1/1, Relational Operator/1
  Constant4/1 -> Relational Operator1/2
  product1/1 -> Relational Operator1/1
  motor_spd_rpm/1 -> Sign/1, Abs2/1
  Switch1/1 -> P/1, Preq/1, Scope/1, Divide4/1, Abs3/1
  torque_req_nm/1 -> Sign1/1, Switch/3, Abs1/1

== system EV_0808_mohu/TM/Intenal Heating ==
  note: 疑问？？
  pwr_loss_w : Inport
  1/thermal resistance : Gain  Gain=tm.thermal_disp_kjpk  SaturateOnIntegerOverflow=on  OutDataTypeStr=Inherit: Same as input  ParamDataTypeStr=Inherit: Same as input
  Add : Sum  Inputs=+-
  Constant2 : Constant  Value=25
  Constant6 : Constant  OutDataTypeStr=Inherit: Inherit via back propagation
  Constant8 : Constant  Value=0
  Discrete Derivative : simulink/Discrete/Discrete Derivative  gainval=1.0  ICPrevScaledInput=tm.init_em_cool_temp_degc  InputProcessing=Inherited  OutMin=[]  OutMax=[]  OutDataType=fixdt(1, 16)  OutScaling=2^-10  DoSatur=off
  Discrete-Time Integrator : DiscreteIntegrator  InitialCondition=tm.init_em_cool_temp_degc  SampleTime=0.01  ICPrevOutput=DiscIntNeverNeededParam  ICPrevScaledInput=DiscIntNeverNeededParam
  Gain : Gain
  Product : Product  Inputs=*/*  SaturateOnIntegerOverflow=on  InputSameDT=on  OutDataTypeStr=Inherit: Same as first input
  Sum2 : Sum  Inputs=+-  SaturateOnIntegerOverflow=on  InputSameDT=on  OutDataTypeStr=Inherit: Same as first input
  Switch3 : Switch  Threshold=tm.max_temp_allowed_degc  SaturateOnIntegerOverflow=on  InputSameDT=on
  coolant heat : Constant  Value=tm.cool_vol_m3*tm.cool_cp_kjpkgk*tm.cool_dens_kgpm3
  cool_temp_degc : Outport  InitialOutput=0
  wires:
  pwr_loss_w/1 -> Product/1
  Discrete-Time Integrator/1 -> Switch3/2, Sum2/1, cool_temp_degc/1
  Switch3/1 -> Discrete-Time Integrator/1
  Constant8/1 -> Switch3/1
  coolant heat/1 -> Product/2
  Constant6/1 -> Product/3
  Sum2/1 -> 1/thermal resistance/1
  Constant2/1 -> Sum2/2
  Product/1 -> Add/1
  1/thermal resistance/1 -> Gain/1
  Add/1 -> Switch3/3
  Gain/1 -> Add/2

== system EV_0808_mohu/TM/Torque management ==
  note: 已改动，疑问解决
  tq_req_nm : Inport
  soc : Inport  Port=2
  cool_temp_degc : Inport  Port=3
  motor_spd_rpm : Inport  Port=4
  Compare To Constant : simulink/Logic and Bit Operations/Compare To Constant  relop=>=  const=0.03  OutDataTypeStr=boolean
  Constant1 : Constant  Value=0
  MinMax : MinMax  Inputs=2
  MinMax1 : MinMax  Function=max  Inputs=2
  Scope : Scope
  Switch : Switch  Criteria=u2 > Threshold
  Switch1 : Switch
  max generation torque : Lookup  InputValues=tm.max_gen_tq_x_rpm  Table=tm.max_gen_tq_y_nm  LookUpMeth=Interpolation-Use End Values
  max motoring torque : Lookup  InputValues=tm.max_mot_tq_x_rpm  Table=tm.max_mot_tq_y_nm  LookUpMeth=Interpolation-Use End Values
  " torque_req_nm" : Outport  InitialOutput=0
  wires:
  Switch1/1 -> Switch/1
  tq_req_nm/1 -> MinMax1/2, MinMax/2, Switch1/2
  soc/1 -> Compare To Constant/1
  Compare To Constant/1 -> Switch/2
  Switch/1 -> " torque_req_nm"/1
  Constant1/1 -> Switch/3
  cool_temp_degc/1 -> Scope/1
  max generation torque/1 -> MinMax1/1
  max motoring torque/1 -> MinMax/1
  motor_spd_rpm/1 -> max generation torque/1, max motoring torque/1
  MinMax/1 -> Switch1/1
  MinMax1/1 -> Switch1/3

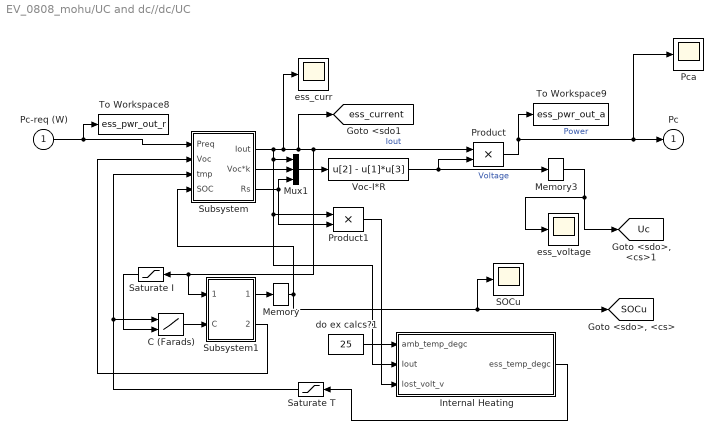
== system EV_0808_mohu/UC and dc//dc/UC ==
  Pc-req (W) : Inport
  C (Farads) : Lookup2D  RowIndex=UC.ess_tmp  ColumnIndex=UC.ess_i  Table=UC.ess_cap  LookUpMeth=Interpolation-Use End Values  SaturateOnIntegerOverflow=on  InputSameDT=on
  Internal Heating : Subsystem
  Memory : Memory  InitialCondition=UC.ess_init_soc
  Memory3 : Memory  InitialCondition=(UC.ess_init_soc*(UC.ess_max_volts-UC.ess_min_volts)+UC.ess_min_volts)*UC.ess_module_num
  Mux1 : Mux  Inputs=3
  Pca : Scope
  Product : Product  SaturateOnIntegerOverflow=on  RndMeth=Zero  InputSameDT=on  OutDataTypeStr=Inherit: Same as first input
  Product1 : Product  SaturateOnIntegerOverflow=on  RndMeth=Zero  InputSameDT=on  OutDataTypeStr=Inherit: Same as first input
  SOCu : Scope
  Saturate I : Saturate  UpperLimit=225  LowerLimit=-225
  Saturate T : Saturate  UpperLimit=40  LowerLimit=0
  Subsystem : Subsystem
  Subsystem1 : Subsystem
  To Workspace8 : ToWorkspace  VariableName=ess_pwr_out_r  SampleTime=-1
  To Workspace9 : ToWorkspace  VariableName=ess_pwr_out_a  SampleTime=-1
  Voc-I*R : Fcn  Expr=u[2] - u[1]*u[3]
  do ex calcs?1 : Constant  Value=25
  ess_curr : Scope
  ess_voltage : Scope
  Pc : Outport  InitialOutput=0
  tag scope: SOCu=global, Uc=global, ess_current=global
  wires:
  Subsystem/1(Iout) -> Internal Heating/2(Iout), Product1/1, Mux1/1, ess_curr/1, [ess_current], Subsystem1/1(Iout), Saturate I/1, Product/1  "Iout"
  Subsystem/3(Rs) -> Product1/2, Mux1/3
  Mux1/1 -> Voc-I*R/1
  Voc-I*R/1 -> Memory3/1, Product/2  "Voltage"
  Saturate I/1 -> C (Farads)/2
  Subsystem/2(Voc*k) -> Mux1/2
  Product/1 -> Pca/1, Pc/1, To Workspace9/1  "Power"
  Subsystem1/1(SOC) -> Memory/1
  Pc-req (W)/1 -> Subsystem/1(Preq), To Workspace8/1
  Saturate T/1 -> Subsystem/3(tmp), C (Farads)/1
  Memory/1 -> SOCu/1, [SOCu], Subsystem/4(SOC)
  C (Farads)/1 -> Subsystem1/2(C)
  do ex calcs?1/1 -> Internal Heating/1(amb_temp_degc)
  Product1/1 -> Internal Heating/3(lost_volt_v)
  Internal Heating/1(ess_temp_degc) -> Saturate T/1
  Memory3/1 -> ess_voltage/1, [Uc]
  Subsystem1/2(VOC) -> Subsystem/2(Voc)

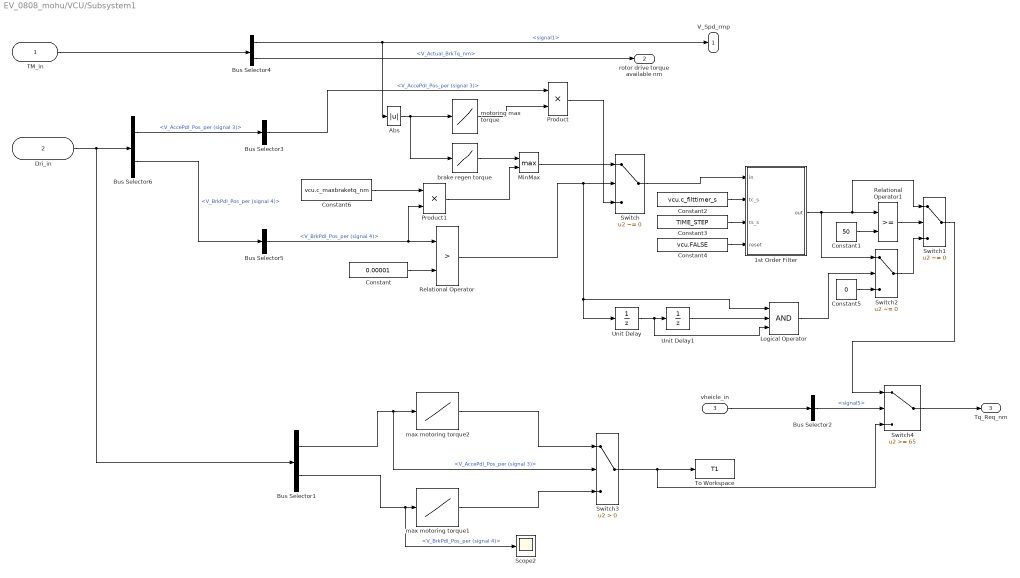
== system EV_0808_mohu/VCU/Subsystem1 ==
  TM_in : Inport
  Dri_in : Inport  Port=2
  vheicle_in : Inport  Port=3
  1st Order Filter : Subsystem
  Abs : Abs
  Bus Selector1 : BusSelector  OutputSignals=V_AccePdl_Pos_per (signal 3),V_BrkPdl_Pos_per (signal 4)
  Bus Selector2 : BusSelector  OutputSignals=signal5
  Bus Selector3 : BusSelector  OutputSignals=V_AccePdl_Pos_per (signal 3)
  Bus Selector4 : BusSelector  OutputSignals=signal1,V_Actual_BrkTq_nm
  Bus Selector5 : BusSelector  OutputSignals=V_BrkPdl_Pos_per (signal 4)
  Bus Selector6 : BusSelector  OutputSignals=V_AccePdl_Pos_per (signal 3),V_BrkPdl_Pos_per (signal 4)
  Constant : Constant  Value=0.00001
  Constant1 : Constant  Value=50
  Constant2 : Constant  Value=vcu.c_filttimer_s
  Constant3 : Constant  Value=TIME_STEP
  Constant4 : Constant  Value=vcu.FALSE  OutDataTypeStr=boolean
  Constant5 : Constant  Value=0
  Constant6 : Constant  Value=vcu.c_maxbraketq_nm
  Logical Operator : Logic  Inputs=3  AllPortsSameDT=off  OutDataTypeStr=boolean
  MinMax : MinMax  Function=max  Inputs=2
  Product : Product  RndMeth=Zero
  Product1 : Product  RndMeth=Zero
  Relational Operator : RelationalOperator  Operator=>  OutDataTypeStr=boolean  RndMeth=Nearest
  Relational Operator1 : RelationalOperator  OutDataTypeStr=boolean  RndMeth=Nearest
  Scope2 : Scope
  Switch : Switch  Criteria=u2 ~= 0
  Switch1 : Switch  Criteria=u2 ~= 0
  Switch2 : Switch  Criteria=u2 ~= 0
  Switch3 : Switch  Criteria=u2 > Threshold
  Switch4 : Switch  Threshold=65
  To Workspace : ToWorkspace  VariableName=T1  SaveFormat=Timeseries  SampleTime=-1
  Unit Delay : UnitDelay  SampleTime=-1
  Unit Delay1 : UnitDelay  SampleTime=-1
  brake regen torque : Lookup  InputValues=tm.max_gen_tq_x_rpm  Table=tm.max_gen_tq_y_nm  LookUpMeth=Interpolation-Use End Values  OutDataTypeStr=single
  max motoring torque1 : Lookup  InputValues=vcu.zd_kaidu  Table=vcu.zd_T  LookUpMeth=Interpolation-Use End Values
  max motoring torque2 : Lookup  InputValues=vcu.qd_kaidu  Table=vcu.qd_T  LookUpMeth=Interpolation-Use End Values
  motoring max torque : Lookup  InputValues=tm.max_mot_tq_x_rpm  Table=tm.max_mot_tq_y_nm  LookUpMeth=Interpolation-Use End Values  OutDataTypeStr=single
  V_Spd_rmp : Outport
  rotor drive torque available nm : Outport  Port=2
  Tq_Req_nm : Outport  Port=3
  wires:
  Bus Selector4/2 -> rotor drive torque available nm/1  "<V_Actual_BrkTq_nm>"
  TM_in/1 -> Bus Selector4/1
  Bus Selector4/1 -> V_Spd_rmp/1, Abs/1  "<signal1>"
  Bus Selector6/2 -> Bus Selector5/1  "<V_BrkPdl_Pos_per (signal 4)>"
  Bus Selector6/1 -> Bus Selector3/1  "<V_AccePdl_Pos_per (signal 3)>"
  Constant5/1 -> Switch2/3
  Switch2/1 -> Switch1/3
  Abs/1 -> motoring max torque/1, brake regen torque/1
  motoring max torque/1 -> Product/2
  Constant/1 -> Relational Operator/2
  Constant6/1 -> Product1/1
  1st Order Filter/1(out) -> Relational Operator1/1, Switch1/1, Switch2/1
  Product/1 -> Switch/3
  Relational Operator1/1 -> Switch1/2
  Constant1/1 -> Relational Operator1/2
  Logical Operator/1 -> Switch2/2
  Unit Delay1/1 -> Logical Operator/2
  Unit Delay/1 -> Unit Delay1/1, Logical Operator/3
  Constant4/1 -> 1st Order Filter/4(reset)
  Constant3/1 -> 1st Order Filter/3(ts_s)
  Constant2/1 -> 1st Order Filter/2(tc_s)
  Switch/1 -> 1st Order Filter/1(in)
  Relational Operator/1 -> Switch/2, Unit Delay/1, Logical Operator/1
  Product1/1 -> MinMax/2
  brake regen torque/1 -> MinMax/1
  MinMax/1 -> Switch/1
  Bus Selector5/1 -> Product1/2, Relational Operator/1  "<V_BrkPdl_Pos_per (signal 4)>"
  Bus Selector3/1 -> Product/1  "<V_AccePdl_Pos_per (signal 3)>"
  Switch1/1 -> Switch4/1
  Bus Selector1/2 -> Scope2/1, max motoring torque1/1  "<V_BrkPdl_Pos_per (signal 4)>"
  max motoring torque1/1 -> Switch3/3
  max motoring torque2/1 -> Switch3/1
  Bus Selector1/1 -> Switch3/2, max motoring torque2/1  "<V_AccePdl_Pos_per (signal 3)>"
  Dri_in/1 -> Bus Selector1/1, Bus Selector6/1
  Switch3/1 -> Switch4/3, To Workspace/1
  Bus Selector2/1 -> Switch4/2  "<signal5>"
  vheicle_in/1 -> Bus Selector2/1
  Switch4/1 -> Tq_Req_nm/1

== system EV_0808_mohu/VCU/Subsystem3 ==
  note: 10000nm/s
  V_Spd_rpm : Inport
  dri_TqReq_nm : Inport  Port=2
  Bus Creator : BusCreator  Inputs=1
  Constant10 : Constant  Value=10000
  Constant7 : Constant  Value=TIME_STEP
  Gain3 : Gain  Gain=-1  ParamDataTypeStr=single  OutDataTypeStr=single
  MinMax1 : MinMax  Function=max  Inputs=2
  MinMax2 : MinMax  Inputs=2
  RateLimit : Subsystem
  max gen torque : Lookup  InputValues=tm.max_gen_tq_x_rpm  Table=tm.max_gen_tq_y_nm  LookUpMeth=Interpolation-Use End Values
  max motoring torque1 : Lookup  InputValues=tm.max_mot_tq_x_rpm  Table=tm.max_mot_tq_y_nm  LookUpMeth=Interpolation-Use End Values
  TM_TqReq_nm : Outport
  wires:
  V_Spd_rpm/1 -> max gen torque/1, max motoring torque1/1
  dri_TqReq_nm/1 -> RateLimit/1(in)
  Gain3/1 -> RateLimit/4(ratelimt_dec)
  Constant10/1 -> RateLimit/3(ratelimt_inc), Gain3/1
  Constant7/1 -> RateLimit/2(steptime)
  Bus Creator/1 -> TM_TqReq_nm/1  "EV_out"
  RateLimit/1(out) -> MinMax1/2
  max gen torque/1 -> MinMax1/1
  max motoring torque1/1 -> MinMax2/1
  MinMax1/1 -> MinMax2/2
  MinMax2/1 -> Bus Creator/1  "tm_tq_req_nm"

== system EV_0808_mohu/VCU/controller ==
  Preq (W) : Inport
  Fuzzy Logic discharge : fuzblock/Fuzzy Logic  Controller  FIS=aaa  OutputSampleNumber=101  DataType=double  FuzzifiedInputs=off  RuleFiringStrengths=off  RuleOutputs=off  AggregatedOutputs=off  SimulateUsing=Interpreted execution  OutOfRangeInputValueMessage=warning  NoRuleFiredMessage=warning  EmptyOutputFuzzySetMessage=warning
  Gain1 : Gain  Gain=1/30000  SaturateOnIntegerOverflow=on  OutDataTypeStr=Inherit: Same as input  ParamDataTypeStr=Inherit: Same as input
  Kb : Scope
  Mux : Mux  Inputs=3
  Pbr : Scope
  Pcr : Scope
  Product : Product  SaturateOnIntegerOverflow=on  RndMeth=Zero  InputSameDT=on  OutDataTypeStr=Inherit: Same as first input
  Sum : Sum  Inputs=|-+  SaturateOnIntegerOverflow=on  InputSameDT=on  OutDataTypeStr=Inherit: Same as first input
  Pb (W) : Outport
  Pc (W) : Outport  Port=2
  wires:
  Mux/1 -> Fuzzy Logic discharge/1
  [SOCb] -> Mux/2
  [SOCu] -> Mux/3
  Gain1/1 -> Mux/1
  Sum/1 -> Pc (W)/1, Pcr/1
  Product/1 -> Pb (W)/1, Pbr/1, Sum/1
  Fuzzy Logic discharge/1 -> Kb/1, Product/1
  Preq (W)/1 -> Sum/2, Product/2, Gain1/1

== system EV_0808_mohu/VCU/续驶里程估计 ==
  batt_in : Inport
  veh_in : Inport  Port=2
  Bus Selector : BusSelector  OutputSignals=V_Volt_v,V_Curr_amp,batt_soc
  Bus Selector1 : BusSelector  OutputSignals=signal5
  Subsystem : Subsystem
  wires:
  batt_in/1 -> Bus Selector/1
  Bus Selector/1 -> [U]  "<V_Volt_v>"
  Bus Selector/3 -> [SOC]  "<batt_soc>"
  Bus Selector/2 -> [I]  "<V_Curr_amp>"
  veh_in/1 -> Bus Selector1/1
  [SOC] -> Subsystem/4(BattSOC)
  [U] -> Subsystem/2(BattVlt)
  [I] -> Subsystem/3(BattCurr)
  Bus Selector1/1 -> Subsystem/1(VehicleSpeed)  "<signal5>"

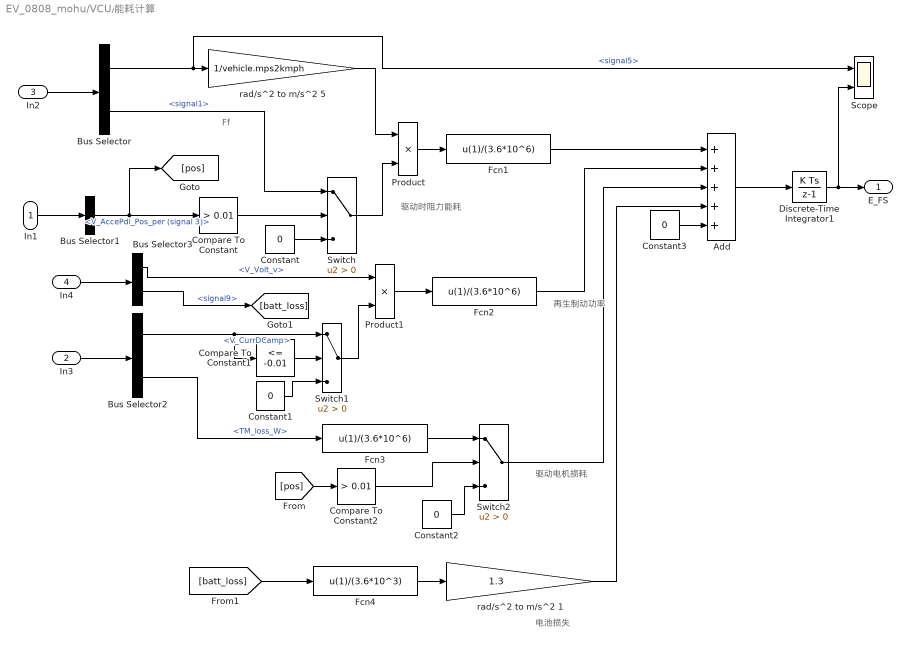
== system EV_0808_mohu/VCU/能耗计算 ==
  note: 驱动电机损耗
  note: Ff
  note: 再生制动功率
  note: 电池损失
  note: 驱动时阻力能耗
  In1 : Inport
  In3 : Inport  Port=2
  In2 : Inport  Port=3
  In4 : Inport  Port=4
  Add : Sum  Inputs=+++++
  Bus Selector : BusSelector  OutputSignals=signal5,signal1
  Bus Selector1 : BusSelector  OutputSignals=V_AccePdl_Pos_per (signal 3)
  Bus Selector2 : BusSelector  OutputSignals=V_CurrDCamp,TM_loss_W
  Bus Selector3 : BusSelector  OutputSignals=V_Volt_v,signal9
  Compare To Constant : simulink/Logic and Bit Operations/Compare To Constant  relop=>  const=0.01  OutDataTypeStr=boolean
  Compare To Constant1 : simulink/Logic and Bit Operations/Compare To Constant  relop=<=  const=-0.01  OutDataTypeStr=boolean
  Compare To Constant2 : simulink/Logic and Bit Operations/Compare To Constant  relop=>  const=0.01  OutDataTypeStr=boolean
  Constant{,1..3} (4 alike) : Constant  Value=0
  Discrete-Time Integrator1 : DiscreteIntegrator  SampleTime=TIME_STEP  LimitOutput=on  LowerSaturationLimit=0  ICPrevOutput=DiscIntNeverNeededParam  ICPrevScaledInput=DiscIntNeverNeededParam
  Fcn1 : Fcn  Expr=u(1)/(3.6*10^6)
  Fcn2 : Fcn  Expr=u(1)/(3.6*10^6)
  Fcn3 : Fcn  Expr=u(1)/(3.6*10^6)
  Fcn4 : Fcn  Expr=u(1)/(3.6*10^3)
  Product : Product
  Product1 : Product
  Scope : Scope  NumInputPorts=2
  Switch : Switch  Criteria=u2 > Threshold
  Switch1 : Switch  Criteria=u2 > Threshold
  Switch2 : Switch  Criteria=u2 > Threshold
  rad/s^2 to m/s^2 1 : Gain  Gain=1.3  SaturateOnIntegerOverflow=on  OutDataTypeStr=Inherit: Same as input  ParamDataTypeStr=Inherit: Same as input
  rad/s^2 to m/s^2 5 : Gain  Gain=1/vehicle.mps2kmph  SaturateOnIntegerOverflow=on  OutDataTypeStr=Inherit: Same as input  ParamDataTypeStr=Inherit: Same as input
  E_FS : Outport
  wires:
  Bus Selector/2 -> Switch/1  "<signal1>"
  Bus Selector/1 -> Scope/1, rad/s^2 to m/s^2 5/1  "<signal5>"
  Switch/1 -> Product/2
  In2/1 -> Bus Selector/1
  Bus Selector1/1 -> [pos], Compare To Constant/1  "<V_AccePdl_Pos_per (signal 3)>"
  Compare To Constant/1 -> Switch/2
  In1/1 -> Bus Selector1/1
  Constant/1 -> Switch/3
  rad/s^2 to m/s^2 5/1 -> Product/1
  Product/1 -> Fcn1/1
  Discrete-Time Integrator1/1 -> Scope/2, E_FS/1
  In3/1 -> Bus Selector2/1
  Bus Selector2/1 -> Compare To Constant1/1, Switch1/1  "<V_CurrDCamp>"
  In4/1 -> Bus Selector3/1
  Product1/1 -> Fcn2/1
  Fcn1/1 -> Add/1
  Fcn2/1 -> Add/2
  Compare To Constant1/1 -> Switch1/2
  Constant1/1 -> Switch1/3
  Add/1 -> Discrete-Time Integrator1/1
  Bus Selector3/1 -> Product1/1  "<V_Volt_v>"
  Switch1/1 -> Product1/2
  Bus Selector2/2 -> Fcn3/1  "<TM_loss_W>"
  Fcn3/1 -> Switch2/1
  Switch2/1 -> Add/3
  [pos] -> Compare To Constant2/1
  Compare To Constant2/1 -> Switch2/2
  Constant2/1 -> Switch2/3
  Bus Selector3/2 -> [batt_loss]  "<signal9>"
  [batt_loss] -> Fcn4/1
  Fcn4/1 -> rad/s^2 to m/s^2 1/1
  Constant3/1 -> Add/5
  rad/s^2 to m/s^2 1/1 -> Add/4

== system EV_0808_mohu/Vehicle/Fbrake ==
  veh_spd_mps : Inport
  brk_pdl_per : Inport  Port=2
  Abs : Abs
  Constant3 : Constant  Value=0.01
  Data Type Conversion : DataTypeConversion
  Dead Zone : DeadZone  LowerValue=-0.01  UpperValue=0.01  SaturateOnIntegerOverflow=on
  Product2 : Product  Inputs=3  SaturateOnIntegerOverflow=on  InputSameDT=on  OutDataTypeStr=Inherit: Same as first input
  Relational Operator : RelationalOperator  OutDataTypeStr=boolean  RndMeth=Nearest
  brake force : Lookup  InputValues=vehicle.brk_tq_x_per  Table=vehicle.brk_tq_y_nm  LookUpMeth=Interpolation-Use End Values
  sign(u) : Lookup  InputValues=[ -0.1 0.1 ]  Table="[-1  1]"  LookUpMeth=Interpolation-Use End Values  OutDataTypeStr=double  SaturateOnIntegerOverflow=on
  Tbrake : Outport  InitialOutput=0
  wires:
  brake force/1 -> Product2/1
  Abs/1 -> Relational Operator/1
  Relational Operator/1 -> Data Type Conversion/1
  Constant3/1 -> Relational Operator/2
  brk_pdl_per/1 -> brake force/1
  veh_spd_mps/1 -> Dead Zone/1, Abs/1
  Dead Zone/1 -> sign(u)/1
  Data Type Conversion/1 -> Product2/3
  sign(u)/1 -> Product2/2
  Product2/1 -> Tbrake/1

== system EV_0808_mohu/Vehicle/Ff ==
  veh_spd_mps : Inport
  Abs : Abs
  Constant1 : Constant  Value=vehicle.tyre_roll_resi_factor
  Constant2 : Constant  Value=vehicle.road_slope_deg
  Constant3 : Constant  Value=0.01
  Data Type Conversion : DataTypeConversion
  Dead Zone : DeadZone  LowerValue=-0.01  UpperValue=0.01  SaturateOnIntegerOverflow=on
  Product1 : Product  SaturateOnIntegerOverflow=on  InputSameDT=on  OutDataTypeStr=Inherit: Same as first input
  Product6 : Product  Inputs=3  SaturateOnIntegerOverflow=on  InputSameDT=on  OutDataTypeStr=Inherit: Same as first input
  Relational Operator : RelationalOperator  OutDataTypeStr=boolean  RndMeth=Nearest
  Rolling resistance : Gain  Gain=vehicle.veh_mass_kg * 9.8  SaturateOnIntegerOverflow=on  OutDataTypeStr=Inherit: Same as input  ParamDataTypeStr=Inherit: Same as input
  Rolling resistance1 : Gain  Gain=3.14/180  SaturateOnIntegerOverflow=on  OutDataTypeStr=Inherit: Same as input  ParamDataTypeStr=Inherit: Same as input
  Trigonometric Function : Trigonometry  Operator=cos
  sign(u) : Lookup  InputValues=[ -0.1 0.1 ]  Table="[-1  1]"  LookUpMeth=Interpolation-Use End Values  OutDataTypeStr=double  SaturateOnIntegerOverflow=on
  Ff : Outport  InitialOutput=0
  wires:
  Constant2/1 -> Rolling resistance1/1
  Rolling resistance1/1 -> Trigonometric Function/1
  Abs/1 -> Relational Operator/1
  Relational Operator/1 -> Data Type Conversion/1
  Constant3/1 -> Relational Operator/2
  Data Type Conversion/1 -> Product6/1
  Rolling resistance/1 -> Product6/2
  Constant1/1 -> Rolling resistance/1
  Trigonometric Function/1 -> Product6/3
  veh_spd_mps/1 -> Dead Zone/1, Abs/1
  Product6/1 -> Product1/2
  Product1/1 -> Ff/1
  sign(u)/1 -> Product1/1
  Dead Zone/1 -> sign(u)/1

== system EV_0808_mohu/Vehicle/Fi ==
  veh_spd_mps : Inport
  Constant2 : Constant  Value=vehicle.road_slope_deg
  Dead Zone : DeadZone  LowerValue=-0.01  UpperValue=0.01  SaturateOnIntegerOverflow=on
  Product1 : Product  SaturateOnIntegerOverflow=on  InputSameDT=on  OutDataTypeStr=Inherit: Same as first input
  Rolling resistance1 : Gain  Gain=3.14/180  SaturateOnIntegerOverflow=on  OutDataTypeStr=Inherit: Same as input  ParamDataTypeStr=Inherit: Same as input
  Rolling resistance2 : Gain  Gain=vehicle.veh_mass_kg * 9.8  SaturateOnIntegerOverflow=on  OutDataTypeStr=Inherit: Same as input  ParamDataTypeStr=Inherit: Same as input
  Trigonometric Function1 : Trigonometry
  sign(u) : Lookup  InputValues=[ -0.1 0.1 ]  Table="[-1  1]"  LookUpMeth=Interpolation-Use End Values  OutDataTypeStr=double  SaturateOnIntegerOverflow=on
  Fi : Outport  InitialOutput=0
  wires:
  Constant2/1 -> Rolling resistance1/1
  Rolling resistance1/1 -> Trigonometric Function1/1
  Trigonometric Function1/1 -> Rolling resistance2/1
  Rolling resistance2/1 -> Product1/2
  sign(u)/1 -> Product1/1
  Dead Zone/1 -> sign(u)/1
  Product1/1 -> Fi/1
  veh_spd_mps/1 -> Dead Zone/1
